simulink model "PanelSubSystem"  (R2022b)
settings: Solver=VariableStepAuto  StartTime=0.0  StopTime=10.0  RelTol=1e-3
undefined symbols (not defined in the file): J, Kd
settings Model: Creator=jprmj  LastModifiedBy=jprmj

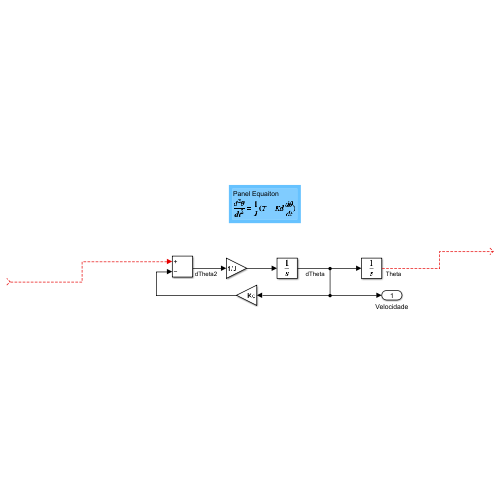
[thumbnail: Simulink's stored preview of the top-level diagram]
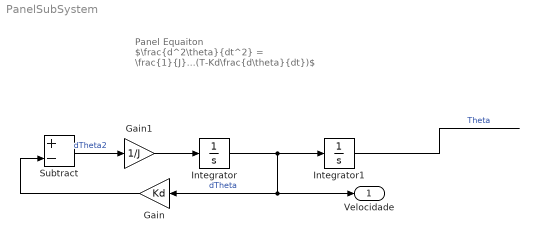
== system PanelSubSystem ==
  note: Panel Equaiton
      | $\frac{d^2\theta}{dt^2} = \frac{1}{J}(T-Kd\frac{d\theta}{dt})$
  Gain : Gain  Gain=Kd
  Gain1 : Gain  Gain=1/J
  Integrator : Integrator
  Integrator1 : Integrator
  Subtract : Sum  Inputs=+-
  Velocidade : Outport
  wires:
  Gain1/1 -> Integrator/1
  ? -> Subtract/1
  Subtract/1 -> Gain1/1  "dTheta2"
  Integrator/1 -> Integrator1/1, Velocidade/1, Gain/1  "dTheta"
  Integrator1/1 -> ?  "Theta"
  Gain/1 -> Subtract/2
